simulink model "robot_echant_etu"  (R2019a)
settings: Solver=VariableStepAuto  StartTime=0.0  StopTime=10.0  RelTol=1e-3
values from neighbouring files (symbols this model uses):
  delta_t = 0.02    [simu_robot_etu.m]
  K = -[-0.6700  -19.9055   -1.0747   -1.9614]    [simu_robot_etu.m]
  ue = 0    [simu_robot_etu.m]
  x0 = [0 pi/10 0 0]'    [simu_robot_etu.m]
  xe = [0 0 0 0]'    [simu_robot_etu.m]
undefined symbols (not defined in the file or in its folder): DiscIntNeverNeededParam
libraries: simulink x1
settings Model: Creator=clotfi  LastModifiedBy=hmoudden

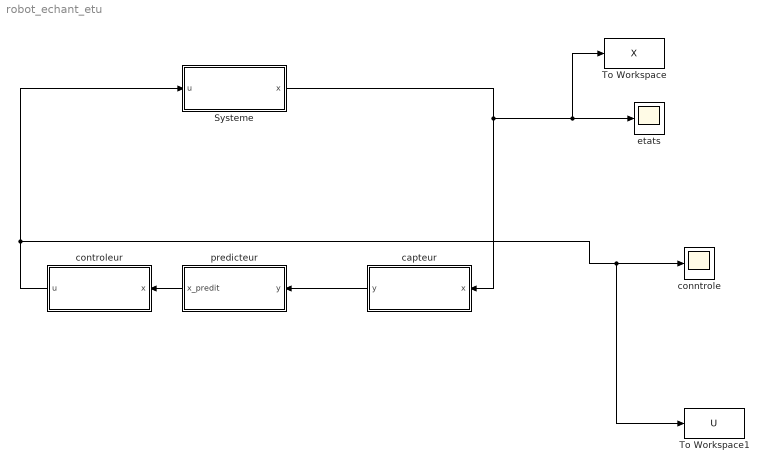
== system robot_echant_etu ==
  "Systeme " : Subsystem
  To Workspace : ToWorkspace  VariableName=X  SaveFormat=Timeseries  SampleTime=-1
  To Workspace1 : ToWorkspace  VariableName=U  SaveFormat=Timeseries  SampleTime=-1
  capteur : Subsystem
  conntrole : Scope
  controleur : Subsystem
  etats : Scope
  predicteur : Subsystem
  wires:
  "Systeme "/1(x) -> To Workspace/1, etats/1, capteur/1(x)
  capteur/1(y) -> predicteur/1(y)
  controleur/1(u) -> "Systeme "/1(u), To Workspace1/1, conntrole/1
  predicteur/1(x_predit) -> controleur/1(x)

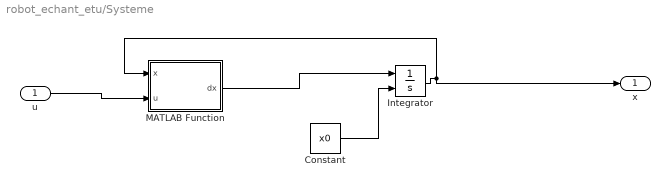
== system robot_echant_etu/Systeme  ==
  u : Inport
  Constant : Constant  Value=x0
  Integrator : Integrator  InitialConditionSource=external  InitialCondition=x0
  MATLAB Function : MATLAB Function  TreatAsAtomicUnit=on
  x : Outport
  wires:
  Integrator/1 -> MATLAB Function/1(x), x/1
  MATLAB Function/1(dx) -> Integrator/1
  u/1 -> MATLAB Function/2(u)
  Constant/1 -> Integrator/2

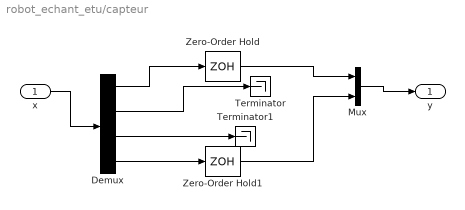
== system robot_echant_etu/capteur ==
  x : Inport
  Demux : Demux
  Mux : Mux  Inputs=2
  Terminator : Terminator
  Terminator1 : Terminator
  Zero-Order Hold : ZeroOrderHold  SampleTime=delta_t
  Zero-Order Hold1 : ZeroOrderHold  SampleTime=delta_t
  y : Outport
  wires:
  x/1 -> Demux/1
  Demux/2 -> Terminator/1
  Demux/3 -> Terminator1/1
  Mux/1 -> y/1
  Demux/4 -> Zero-Order Hold1/1
  Demux/1 -> Zero-Order Hold/1
  Zero-Order Hold/1 -> Mux/1
  Zero-Order Hold1/1 -> Mux/2

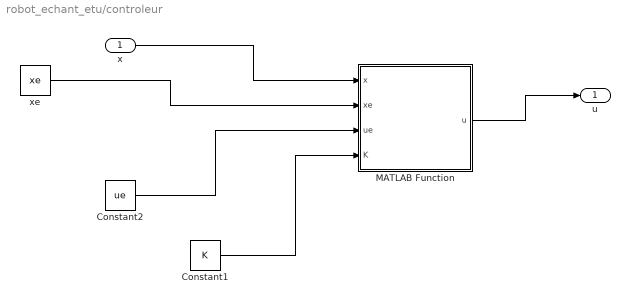
== system robot_echant_etu/controleur ==
  x : Inport
  Constant1 : Constant  Value=K
  Constant2 : Constant  Value=ue
  MATLAB Function : MATLAB Function  TreatAsAtomicUnit=on
  xe : Constant  Value=xe
  u : Outport
  wires:
  x/1 -> MATLAB Function/1(x)
  xe/1 -> MATLAB Function/2(xe)
  Constant1/1 -> MATLAB Function/4(K)
  Constant2/1 -> MATLAB Function/3(ue)
  MATLAB Function/1(u) -> u/1

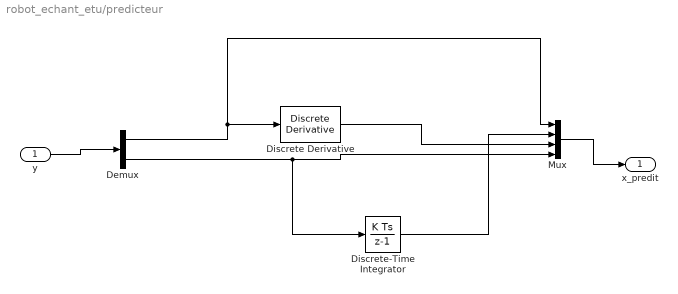
== system robot_echant_etu/predicteur ==
  y : Inport
  Demux : Demux  Outputs=2
  Discrete Derivative : simulink/Discrete/Discrete Derivative  gainval=1.0  ICPrevScaledInput=0.0  OutMin=[]  OutMax=[]  OutDataType=fixdt(1, 16)  OutScaling=2^-10  DoSatur=off
  Discrete-Time Integrator : DiscreteIntegrator  InitialCondition=x0(3)  SampleTime=-1  ICPrevOutput=DiscIntNeverNeededParam  ICPrevScaledInput=DiscIntNeverNeededParam
  Mux : Mux
  x_predit : Outport
  wires:
  Mux/1 -> x_predit/1
  y/1 -> Demux/1
  Demux/1 -> Discrete Derivative/1, Mux/1
  Demux/2 -> Discrete-Time Integrator/1, Mux/4
  Discrete Derivative/1 -> Mux/3
  Discrete-Time Integrator/1 -> Mux/2

== matlab function robot_echant_etu/Systeme /MATLAB Function ==
  data: x input; u input; dx output
function dx   = fonction( x, u)
%   Dynamic equations of motion of the segway on an axis.
%   Inputs: - x = [theta psi dtheta dpsi]
%               theta: average angle of the wheels      [rad]
%               psi: body pitch angle                   [rad]
%               dtheta: average velocity of the wheels  [rad/s]
%               dpsi: body pitch velocity               [rad/s]
%          - u: DC motor voltage (same value for both motors) [V]

    % State
    psi = x(2);
    dtheta = x(3);
    dpsi = x(4);

    % Parameters
    
    g = 9.81;           % gravity acceleration [m/sec^2]
    m = 0.03;           % wheel weight [kg]
    R = 0.04;           % wheel radius [m]
    Jw = m*R^2/2;       % wheel inertia moment [kg*m^2]
    M = 0.6;            % body weight [kg]
    H = 0.144;          % body height [m]
    L = H/2;            % distance of the center of mass from the wheel axle [m]
    Jpsi = M*L^2/3;     % body pitch inertia [kgm^2]
    Jm = 1e-5;          % DC motor inertia moment [kgm^2]
    Rm = 6.69;          % DC motor resistance [Ohm]
    Kb = 0.468;         % DC motor back EMF constant [Vsec/rad]
    Kt = 0.317;         % DC motor torque constant [Nm/A]
    n = 1;              % gear ratio
    fm = 0.0022;        % friction coefficient between body and DC motor
    fw = 0;             % friction coefficient between wheel and floor
    
    % Equations of motion
    c1 = (2*m+M)*R^2 + 2*Jw + 2*n^2*Jm;
    c2 = M*L*R*cos(psi) - 2*n^2*Jm;
    c3 = -M*L*R*dpsi^2*sin(psi);
    c4 = M*L^2 + Jpsi + 2*n^2*Jm;
    c5 = -M*g*L*sin(psi);

    alpha = Kt/Rm;
    beta = Kt*Kb/Rm + fm;

    Ftheta = alpha*(2*u) - 2*(beta+fw)*dtheta + 2*beta*dpsi;
    Fpsi = -alpha*(2*u) + 2*beta*dtheta - 2*beta*dpsi;

    ddtheta = (c4*c3 - c2*c5 + c4*Ftheta - c2*Fpsi)/(c4*c1 - c2^2);
    ddpsi = (Fpsi- c2*ddtheta - c5)/c4;
    dx = [dtheta dpsi ddtheta ddpsi]';

end

== matlab function robot_echant_etu/controleur/MATLAB Function ==
  data: x input; u output; xe input; ue input; K input
function u = fcn(x,xe,ue,K)
 u = ue+ K(:)'*( x(:)-xe(:));
end
